simulink model "SEPIC_uniform_shading_mppt"  (R2021b)
settings: Solver=ode15s  StartTime=0.0  StopTime=1  FixedStep=1e-6  MaxStep=1e-5  RelTol=1e-3
libraries: spsDiodeLib x57, spsPVArrayLib x49, spsSeriesRLCBranchLib x6, spsMeanLib x6, spsCurrentMeasurementLib x2, spsVoltageMeasurementLib x2, simulink x1, spsIGBTDiodeLib x1, spspowerguiLib x1
settings Model: Creator=Vishal  LastModifiedBy=Vishal
settings DataIOCC: ReturnWorkspaceOutputs=off

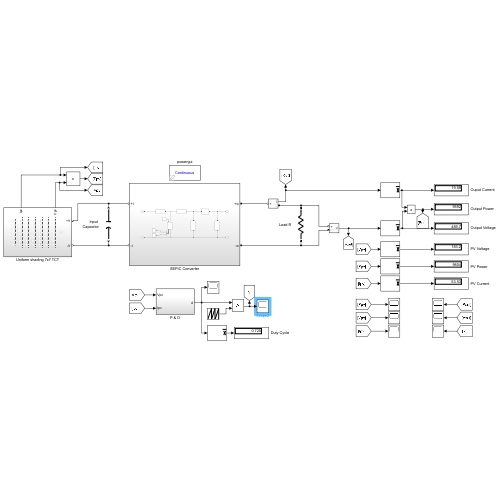
[thumbnail: Simulink's stored preview of the top-level diagram]
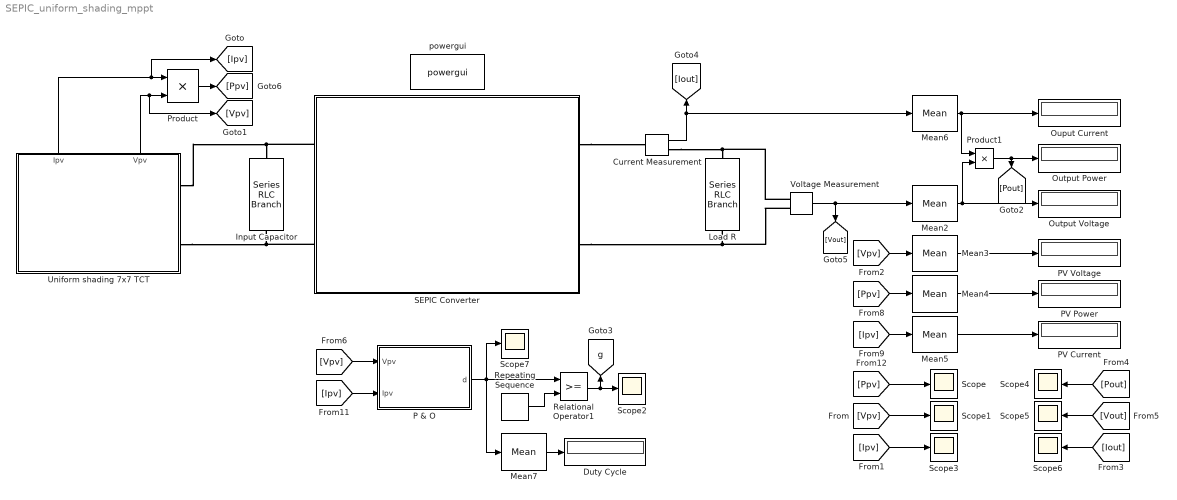
== system SEPIC_uniform_shading_mppt ==
  Current Measurement : spsCurrentMeasurementLib/Current Measurement  PhasorSimulation=off  OutputType=Complex  PSBequivalent=0
  Duty Cycle : Display
  Input Capacitor : spsSeriesRLCBranchLib/Series RLC Branch  LConnTagsString=__new0  RConnTagsString=__new0  BranchType=C  Resistance=1e-4  Inductance=1e-3  SetiL0=off  InitialCurrent=0  Capacitance=1e-3  Setx0=off  InitialVoltage=0  Measurements=None
  Load R : spsSeriesRLCBranchLib/Series RLC Branch  LConnTagsString=__new0  RConnTagsString=__new0  BranchType=R  Resistance=25  Inductance=1e-3  SetiL0=off  InitialCurrent=0  Capacitance=1e-6  Setx0=off  InitialVoltage=0  Measurements=None
  Mean{2..7} (6 alike) : spsMeanLib/Mean  Freq=10000  Vinit=0  Ts=0
  Ouput Current : Display
  Output Power : Display
  Output Voltage : Display
  P & O : Subsystem
  PV Current : Display
  PV Power : Display
  PV Voltage : Display
  Product : Product
  Product1 : Product
  Relational Operator1 : RelationalOperator  OutDataTypeStr=boolean  RndMeth=Simplest
  Repeating Sequence : simulink/Sources/Repeating Sequence  rep_seq_t=[0 1/10000]  rep_seq_y=[0 1]
  SEPIC Converter : Subsystem
  Scope{,1..7} (8 alike) : Scope
  Uniform shading 7x7 TCT : Subsystem
      settings: PortSchema="{\"entries\":[{\"content\":{\"sides\":[{\"content\":{\"connectorIds\":[]},\"type\":\"ConnectorPlacement.EquallySpacedRectSide\",\"uuid\":\"2b1d5fe4-4caa-4b35-804e-a42f89d402b6\"},{\"content\":{\"connectorIds\":[\"RConn1\",\"RConn2\"],\"side\":\"RIGHT\"},\"type\":\"ConnectorPlacement.EquallySpacedRectSide\",\"uuid\":\"1cc3aab2-123e-49fa-87cd-798c1955a822\"},{\"content\":{\"connectorIds\":[\"Out1\",\"Out2\"],\"side\":\"TOP\"},\"type\":\"ConnectorPlacement.EquallySpacedRectSide\",\"uuid\":\"89cee466-e232-436a-aff0-a5a0928aa5af\"}]},\"type\":\"ConnectorPlacement.EquallySpacedConnector\",\"uuid\":\"4c42cdc2-2679-4c70-9c6c-b31cb19848fa\"}],\"packageUris\":[\"http://schema.mathworks.com/mf0/Connector/R2020b\"],\"version\":\"1.0\"}"
  Voltage Measurement : spsVoltageMeasurementLib/Voltage Measurement  PhasorSimulation=off  OutputType=Complex  PSBequivalent=0
  powergui : spspowerguiLib/powergui  Priority=1  SimulationMode=Continuous  SampleTime=1e-6  frequency=60  Iterations=50  frequencyindice=0  Pbase=100e6  ErrMax=1e-4  UnitsV=kV  UnitsW=MW  buscounter=0  FunctionMessages=off  echomessages=off  EnableUseOfTLC=off  CurrentSourceSwitches=off  DisableSnubberDevices=off  DisableRonSwitches=off  DisableVfSwitches=off  DisplayEquations=off  AutomaticDiscreteSolvers=off  SolverType=Tustin/Backward Euler (TBE)  Interpol=off  ExternalGateDelay=off  methode=off  Ts=100  x0status=blocks  SPID=on  SwTol=0  HookPort=off  NonlinearTolerance=1e-4  nMaxIteration=100  ContinueOnMaxIteration=off  RestoreLinks=warning  ResistiveCurrentMeasurement=off  Frange=[0:2:500]  Ylog=off  Xlog=on  ShowGrid=off  save=off  variable=ZData  structure=0  ZoomFFT=off  StartTime=0.0  cycles=1  DisplayStyle=1  fundamental=60  FreqAxis=off  MaxFrequency=1000  frequencyindicesteady=1  RmsSteady=1  display=off
  tag scope: g=global
  wires:
  Product/1 -> [Ppv]
  Uniform shading 7x7 TCT/2(Vpv) -> [Vpv], Product/2
  Uniform shading 7x7 TCT/1(Ipv) -> [Ipv], Product/1
  P & O/1(d) -> Mean7/1, Scope7/1, Relational Operator1/1
  Mean7/1 -> Duty Cycle/1
  [Ppv] -> Scope/1
  Repeating Sequence/1 -> Relational Operator1/2
  [Pout] -> Scope4/1
  [Vout] -> Scope5/1
  [Ipv] -> Mean5/1
  [Iout] -> Scope6/1
  [Ipv] -> Scope3/1
  Relational Operator1/1 -> Scope2/1, [g]
  [Vpv] -> P & O/1(Vpv)
  Product1/1 -> Output Power/1, [Pout]
  [Ppv] -> Mean4/1
  [Ipv] -> P & O/2(Ipv)
  [Vpv] -> Mean3/1
  Mean6/1 -> Ouput Current/1, Product1/1
  Mean2/1 -> Output Voltage/1, Product1/2
  Mean4/1 -> PV Power/1
  Mean3/1 -> PV Voltage/1
  Mean5/1 -> PV Current/1
  Current Measurement/1 -> [Iout], Mean6/1
  [Vpv] -> Scope1/1
  Voltage Measurement/1 -> Mean2/1, [Vout]
  connections:
  Input Capacitor/LConn1 -- SEPIC Converter/LConn1 -- Uniform shading 7x7 TCT/RConn1
  Input Capacitor/RConn1 -- SEPIC Converter/LConn2 -- Uniform shading 7x7 TCT/RConn2
  Current Measurement/RConn1 -- Voltage Measurement/LConn1 -- Load R/LConn1
  Voltage Measurement/LConn2 -- SEPIC Converter/RConn2 -- Load R/RConn1
  SEPIC Converter/RConn1 -- Current Measurement/LConn1

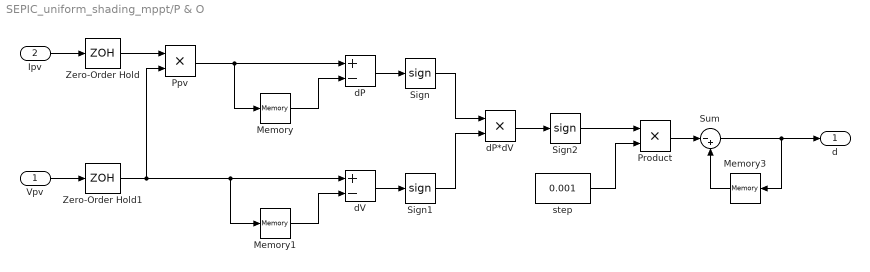
== system SEPIC_uniform_shading_mppt/P & O ==
  Vpv : Inport
  Ipv : Inport  Port=2
  Memory : Memory  InheritSampleTime=on
  Memory1 : Memory  InheritSampleTime=on
  Memory3 : Memory  InitialCondition=0.5  InheritSampleTime=on
  Ppv : Product  RndMeth=Zero
  Product : Product  RndMeth=Zero
  Sign : Signum
  Sign1 : Signum
  Sign2 : Signum
  Sum : Sum  Inputs=|-+
  Zero-Order Hold : ZeroOrderHold  SampleTime=0.002
  Zero-Order Hold1 : ZeroOrderHold  SampleTime=0.002
  dP : Sum  Inputs=+-
  dP*dV : Product  RndMeth=Zero
  dV : Sum  Inputs=+-
  step : Constant  Value=0.001
  d : Outport
  wires:
  Memory1/1 -> dV/2
  Memory/1 -> dP/2
  Vpv/1 -> Zero-Order Hold1/1
  dV/1 -> Sign1/1
  step/1 -> Product/2
  Product/1 -> Sum/1
  Sign/1 -> dP*dV/1
  Sign1/1 -> dP*dV/2
  dP*dV/1 -> Sign2/1
  Ipv/1 -> Zero-Order Hold/1
  Zero-Order Hold1/1 -> dV/1, Memory1/1, Ppv/2
  Zero-Order Hold/1 -> Ppv/1
  Ppv/1 -> Memory/1, dP/1
  dP/1 -> Sign/1
  Sign2/1 -> Product/1
  Sum/1 -> d/1, Memory3/1
  Memory3/1 -> Sum/2

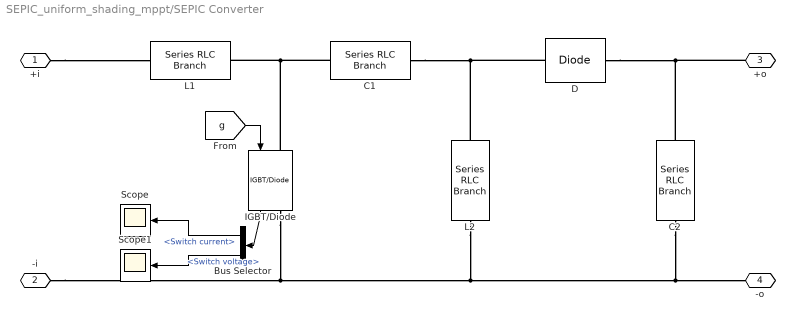
== system SEPIC_uniform_shading_mppt/SEPIC Converter ==
  Bus Selector : BusSelector  OutputSignals=Switch current,Switch voltage
  C1 : spsSeriesRLCBranchLib/Series RLC Branch  LConnTagsString=__new0  RConnTagsString=__new0  BranchType=C  Resistance=1  Inductance=1e-3  SetiL0=off  InitialCurrent=0  Capacitance=5.7143e-04  Setx0=off  InitialVoltage=0  Measurements=None
  C2 : spsSeriesRLCBranchLib/Series RLC Branch  LConnTagsString=__new0  RConnTagsString=__new0  BranchType=C  Resistance=1  Inductance=1e-3  SetiL0=off  InitialCurrent=0  Capacitance=0.0029  Setx0=off  InitialVoltage=0  Measurements=None
  D : spsDiodeLib/Diode  Ron=0.001  Lon=0  Vf=0  IC=0  UseSnubber=0  Rs=500  Cs=250e-9  Measurements=off
  IGBT/Diode : spsIGBTDiodeLib/IGBT//Diode  Ron=1e-3  Rs=1e5  Cs=inf  Measurements=on
  L1 : spsSeriesRLCBranchLib/Series RLC Branch  LConnTagsString=__new0  RConnTagsString=__new0  BranchType=L  Resistance=1  Inductance=0.0143  SetiL0=off  InitialCurrent=0  Capacitance=1e-6  Setx0=off  InitialVoltage=0  Measurements=None
  L2 : spsSeriesRLCBranchLib/Series RLC Branch  LConnTagsString=__new0  RConnTagsString=__new0  BranchType=L  Resistance=1  Inductance=0.0107  SetiL0=off  InitialCurrent=0  Capacitance=1e-6  Setx0=off  InitialVoltage=0  Measurements=None
  Scope : Scope
  Scope1 : Scope
  +i : PMIOPort  Side=Left
  -i : PMIOPort  Port=2  Side=Left
  +o : PMIOPort  Port=3  Side=Right
  -o : PMIOPort  Port=4  Side=Right
  wires:
  [g] -> IGBT/Diode/1
  Bus Selector/1 -> Scope/1  "<Switch current>"
  IGBT/Diode/1 -> Bus Selector/1
  Bus Selector/2 -> Scope1/1  "<Switch voltage>"
  connections:
  C1/LConn1 -- L1/RConn1 -- IGBT/Diode/LConn1
  C1/RConn1 -- L2/RConn1 -- D/LConn1
  C2/LConn1 -- D/RConn1 -- +o/RConn1
  +i/RConn1 -- L1/LConn1
  -i/RConn1 -- L2/LConn1 -- -o/RConn1 -- C2/RConn1 -- IGBT/Diode/RConn1

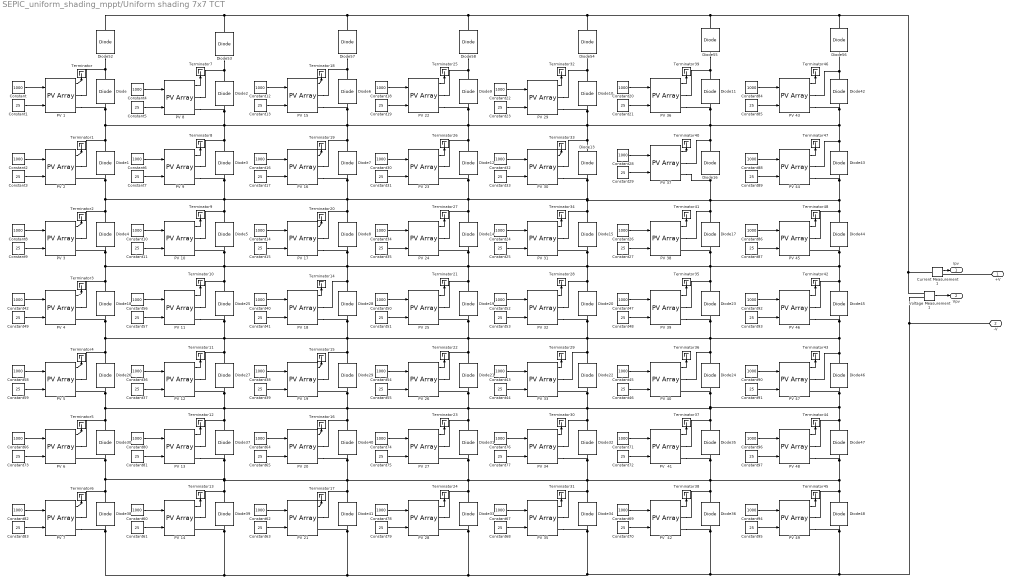
== system SEPIC_uniform_shading_mppt/Uniform shading 7x7 TCT ==
  Constant{,2,4,6,8,10,12,14,16,18,20,22,24,26,28,30,32,34,36,38,40,42..43,45,47,50,52,54,56,58,60,62,64,66..67,69,71,74,76,78,80,82,84,86,88,90,92,94,96} (49 alike) : Constant  Value=1000
  Constant{1,3,5,7,9,11,13,15,17,19,21,23,25,27,29,31,33,35,37,39,41,44,46,48..49,51,53,55,57,59,61,63,65,68,70,72..73,75,77,79,81,83,85,87,89,91,93,95,97} (49 alike) : Constant  Value=25
  Current Measurement1 : spsCurrentMeasurementLib/Current Measurement  PhasorSimulation=off  OutputType=Complex  PSBequivalent=0
  Diode{,1..48,52..58} (56 alike) : spsDiodeLib/Diode  Ron=0.001  Lon=0  Vf=0  IC=0  UseSnubber=0  Rs=500  Cs=250e-9  Measurements=off
  PV  41 : spsPVArrayLib/PV Array  Npar=1  Nser=1  PlotType=array @ 1000 W/m2 & specified temperatures  S_vec="[ 1000  500  100 ]"  Temp_C_vec="[ 45 25  ]"  ModuleName=Kyocera Solar KC200GT  PlotWhenSelected=off  Pm=200.143  Ncell=54  Voc=32.9  Isc=8.21  Vm=26.3  Im=7.61  beta_Voc_pc=-0.355  alpha_Isc_pc=0.06  beta_Voc=-0.11679  alpha_Isc=0.004926  IL=8.2288  I0=2.3234e-10  nI=0.97734  Rsh=150.6844  Rs=0.34484  RobustModel=off  RobustCellTemperature=313.3991  BAL=on  Tc=1e-6  Tfilter=5e-5
  PV  42 : spsPVArrayLib/PV Array  Npar=1  Nser=1  PlotType=array @ 1000 W/m2 & specified temperatures  S_vec="[ 1000  500  100 ]"  Temp_C_vec="[ 45 25  ]"  ModuleName=Kyocera Solar KC200GT  PlotWhenSelected=off  Pm=200.143  Ncell=54  Voc=32.9  Isc=8.21  Vm=26.3  Im=7.61  beta_Voc_pc=-0.355  alpha_Isc_pc=0.06  beta_Voc=-0.11679  alpha_Isc=0.004926  IL=8.2288  I0=2.3234e-10  nI=0.97734  Rsh=150.6844  Rs=0.34484  RobustModel=off  RobustCellTemperature=313.3991  BAL=on  Tc=1e-6  Tfilter=5e-5
  PV {1..40,43..49} (47 alike) : spsPVArrayLib/PV Array  Npar=1  Nser=1  PlotType=array @ 1000 W/m2 & specified temperatures  S_vec="[ 1000  500  100 ]"  Temp_C_vec="[ 45 25  ]"  ModuleName=Kyocera Solar KC200GT  PlotWhenSelected=off  Pm=200.143  Ncell=54  Voc=32.9  Isc=8.21  Vm=26.3  Im=7.61  beta_Voc_pc=-0.355  alpha_Isc_pc=0.06  beta_Voc=-0.11679  alpha_Isc=0.004926  IL=8.2288  I0=2.3234e-10  nI=0.97734  Rsh=150.6844  Rs=0.34484  RobustModel=off  RobustCellTemperature=313.3991  BAL=on  Tc=1e-6  Tfilter=5e-5
  Terminator{,1..48} (49 alike) : Terminator
  Voltage Measurement1 : spsVoltageMeasurementLib/Voltage Measurement  PhasorSimulation=off  OutputType=Complex  PSBequivalent=0
  +V : PMIOPort  Side=Right
  -V : PMIOPort  Port=2  Side=Right
  Ipv : Outport
  Vpv : Outport  Port=2
  wires:
  Constant91/1 -> PV 47/2
  PV 20/1 -> Terminator16/1
  Constant93/1 -> PV 46/2
  PV 23/1 -> Terminator26/1
  Constant87/1 -> PV 45/2
  Constant46/1 -> PV 40/2
  PV 49/1 -> Terminator45/1
  PV 47/1 -> Terminator43/1
  PV 48/1 -> Terminator44/1
  Constant60/1 -> PV 14/1
  Constant70/1 -> PV  42/2
  Constant1/1 -> PV 1/2
  Constant61/1 -> PV 14/2
  PV  41/1 -> Terminator37/1
  PV 11/1 -> Terminator10/1
  Constant8/1 -> PV 3/1
  Constant39/1 -> PV 19/2
  Constant47/1 -> PV 39/1
  Constant73/1 -> PV 6/2
  Constant25/1 -> PV 31/2
  Constant33/1 -> PV 30/2
  PV 30/1 -> Terminator33/1
  PV 45/1 -> Terminator48/1
  Constant13/1 -> PV 15/2
  Constant86/1 -> PV 45/1
  Constant6/1 -> PV 9/1
  PV 27/1 -> Terminator23/1
  Constant82/1 -> PV 7/1
  PV 22/1 -> Terminator25/1
  Constant58/1 -> PV 5/1
  PV 35/1 -> Terminator31/1
  Constant74/1 -> PV 27/1
  PV 1/1 -> Terminator/1
  Constant32/1 -> PV 30/1
  Constant55/1 -> PV 26/2
  PV  42/1 -> Terminator38/1
  PV 28/1 -> Terminator24/1
  Constant65/1 -> PV 20/2
  Constant50/1 -> PV 25/1
  Constant40/1 -> PV 18/1
  Constant37/1 -> PV 12/2
  Constant90/1 -> PV 47/1
  PV 7/1 -> Terminator6/1
  PV 6/1 -> Terminator5/1
  Constant/1 -> PV 1/1
  PV 36/1 -> Terminator39/1
  PV 29/1 -> Terminator32/1
  PV 2/1 -> Terminator1/1
  Constant94/1 -> PV 49/1
  Constant22/1 -> PV 29/1
  Constant38/1 -> PV 19/1
  Constant16/1 -> PV 16/1
  PV 46/1 -> Terminator42/1
  PV 9/1 -> Terminator8/1
  Constant48/1 -> PV 39/2
  PV 10/1 -> Terminator9/1
  Constant88/1 -> PV 44/1
  Constant11/1 -> PV 10/2
  Constant54/1 -> PV 26/1
  Constant56/1 -> PV 11/1
  Constant69/1 -> PV  42/1
  PV 44/1 -> Terminator47/1
  Constant20/1 -> PV 36/1
  PV 34/1 -> Terminator30/1
  Constant83/1 -> PV 7/2
  Constant27/1 -> PV 38/2
  PV 43/1 -> Terminator46/1
  Constant23/1 -> PV 29/2
  Constant31/1 -> PV 23/2
  Constant9/1 -> PV 3/2
  Constant28/1 -> PV 37/1
  PV 4/1 -> Terminator3/1
  Constant30/1 -> PV 23/1
  Constant79/1 -> PV 28/2
  Constant49/1 -> PV 4/2
  PV 12/1 -> Terminator11/1
  Constant5/1 -> PV 8/2
  PV 18/1 -> Terminator14/1
  Constant96/1 -> PV 48/1
  PV 39/1 -> Terminator35/1
  Constant97/1 -> PV 48/2
  Constant89/1 -> PV 44/2
  Constant53/1 -> PV 32/2
  Constant2/1 -> PV 2/1
  Constant64/1 -> PV 20/1
  Constant72/1 -> PV  41/2
  PV 15/1 -> Terminator18/1
  Constant26/1 -> PV 38/1
  PV 38/1 -> Terminator41/1
  Constant45/1 -> PV 40/1
  PV 8/1 -> Terminator7/1
  PV 17/1 -> Terminator20/1
  Constant57/1 -> PV 11/2
  PV 14/1 -> Terminator13/1
  Constant43/1 -> PV 33/1
  Constant19/1 -> PV 22/2
  PV 24/1 -> Terminator27/1
  Constant35/1 -> PV 24/2
  Constant59/1 -> PV 5/2
  Constant84/1 -> PV 43/1
  PV 32/1 -> Terminator28/1
  Constant67/1 -> PV 35/1
  PV 40/1 -> Terminator36/1
  PV 19/1 -> Terminator15/1
  PV 33/1 -> Terminator29/1
  PV 13/1 -> Terminator12/1
  Constant17/1 -> PV 16/2
  Constant10/1 -> PV 10/1
  Voltage Measurement1/1 -> Vpv/1
  Constant21/1 -> PV 36/2
  PV 5/1 -> Terminator4/1
  Constant66/1 -> PV 6/1
  Constant85/1 -> PV 43/2
  Constant51/1 -> PV 25/2
  Constant52/1 -> PV 32/1
  Constant81/1 -> PV 13/2
  Constant36/1 -> PV 12/1
  Constant44/1 -> PV 33/2
  Constant42/1 -> PV 4/1
  PV 16/1 -> Terminator19/1
  PV 26/1 -> Terminator22/1
  Constant14/1 -> PV 17/1
  PV 31/1 -> Terminator34/1
  PV 3/1 -> Terminator2/1
  Constant4/1 -> PV 8/1
  Constant41/1 -> PV 18/2
  Constant92/1 -> PV 46/1
  Constant80/1 -> PV 13/1
  Constant63/1 -> PV 21/2
  Constant3/1 -> PV 2/2
  Constant77/1 -> PV 34/2
  Constant24/1 -> PV 31/1
  PV 37/1 -> Terminator40/1
  Constant71/1 -> PV  41/1
  Constant95/1 -> PV 49/2
  Constant29/1 -> PV 37/2
  Constant34/1 -> PV 24/1
  Constant76/1 -> PV 34/1
  Constant75/1 -> PV 27/2
  Constant15/1 -> PV 17/2
  Constant78/1 -> PV 28/1
  PV 25/1 -> Terminator21/1
  Constant18/1 -> PV 22/1
  Constant68/1 -> PV 35/2
  Constant7/1 -> PV 9/2
  Constant12/1 -> PV 15/1
  Constant62/1 -> PV 21/1
  PV 21/1 -> Terminator17/1
  Current Measurement1/1 -> Ipv/1
  connections:
  PV 7/RConn1 -- PV 13/RConn2 -- Diode37/LConn1 -- PV 20/RConn2 -- Diode40/LConn1 -- PV 28/RConn1 -- Diode33/RConn1 -- PV 34/RConn2 -- Diode32/LConn1 -- PV  41/RConn2 -- Diode35/LConn1 -- Diode47/LConn1 -- PV 48/RConn2 -- Diode48/RConn1 -- PV 49/RConn1 -- Diode36/RConn1 -- PV  42/RConn1 -- Diode34/RConn1 -- PV 35/RConn1 -- PV 27/RConn2 -- Diode31/LConn1 -- Diode41/RConn1 -- PV 21/RConn1 -- Diode39/RConn1 -- PV 14/RConn1 -- Diode30/LConn1 -- PV 6/RConn2 -- Diode38/RConn1
  PV 22/RConn1 -- Diode9/RConn1 -- Diode58/LConn1
  Diode54/RConn1 -- Diode53/RConn1 -- Diode52/RConn1 -- Diode57/RConn1 -- Diode58/RConn1 -- Diode55/RConn1 -- Current Measurement1/LConn1 -- Voltage Measurement1/LConn1 -- Diode56/RConn1
  Diode4/LConn1 -- Diode18/RConn1 -- PV 4/RConn1 -- PV 11/RConn1 -- Diode25/RConn1 -- PV 18/RConn1 -- Diode28/RConn1 -- PV 39/RConn1 -- Diode23/RConn1 -- Diode45/RConn1 -- PV 46/RConn1 -- Diode44/LConn1 -- PV 45/RConn2 -- Diode17/LConn1 -- PV 38/RConn2 -- Diode15/LConn1 -- PV 31/RConn2 -- PV 32/RConn1 -- Diode20/RConn1 -- PV 25/RConn1 -- Diode19/RConn1 -- PV 24/RConn2 -- Diode14/LConn1 -- Diode8/LConn1 -- PV 17/RConn2 -- Diode5/LConn1 -- PV 10/RConn2 -- PV 3/RConn2
  Voltage Measurement1/LConn2 -- -V/RConn1 -- Diode48/LConn1 -- PV 49/RConn2 -- Diode33/LConn1 -- PV 28/RConn2 -- Diode41/LConn1 -- PV 21/RConn2 -- Diode39/LConn1 -- PV 14/RConn2 -- Diode38/LConn1 -- PV 7/RConn2 -- Diode34/LConn1 -- PV 35/RConn2 -- Diode36/LConn1 -- PV  42/RConn2
  PV 15/RConn1 -- Diode6/RConn1 -- Diode57/LConn1
  PV 1/RConn1 -- Diode/RConn1 -- Diode52/LConn1
  PV 8/RConn1 -- Diode2/RConn1 -- Diode53/LConn1
  PV 29/RConn1 -- Diode10/RConn1 -- Diode54/LConn1
  PV 5/RConn2 -- Diode30/RConn1 -- PV 6/RConn1 -- Diode27/LConn1 -- PV 12/RConn2 -- PV 13/RConn1 -- Diode37/RConn1 -- PV 19/RConn2 -- Diode29/LConn1 -- Diode40/RConn1 -- PV 20/RConn1 -- Diode21/LConn1 -- PV 26/RConn2 -- PV 27/RConn1 -- Diode31/RConn1 -- Diode46/LConn1 -- PV 47/RConn2 -- Diode47/RConn1 -- PV 48/RConn1 -- Diode24/LConn1 -- PV 40/RConn2 -- PV  41/RConn1 -- Diode35/RConn1 -- Diode22/LConn1 -- PV 33/RConn2 -- PV 34/RConn1 -- Diode32/RConn1 -- Diode26/LConn1
  PV 43/RConn1 -- Diode56/LConn1 -- Diode42/RConn1
  PV 3/RConn1 -- Diode4/RConn1 -- Diode8/RConn1 -- PV 17/RConn1 -- PV 23/RConn2 -- Diode12/LConn1 -- Diode13/LConn1 -- PV 30/RConn2 -- PV 37/RConn2 -- Diode16/LConn1 -- Diode43/LConn1 -- PV 44/RConn2 -- Diode44/RConn1 -- PV 45/RConn1 -- Diode17/RConn1 -- PV 38/RConn1 -- PV 31/RConn1 -- Diode15/RConn1 -- PV 24/RConn1 -- Diode14/RConn1 -- PV 16/RConn2 -- Diode7/LConn1 -- Diode5/RConn1 -- PV 10/RConn1 -- PV 9/RConn2 -- Diode3/LConn1 -- PV 2/RConn2 -- Diode1/LConn1
  PV 5/RConn1 -- PV 19/RConn1 -- Diode29/RConn1 -- PV 25/RConn2 -- Diode19/LConn1 -- Diode20/LConn1 -- PV 32/RConn2 -- Diode23/LConn1 -- PV 39/RConn2 -- PV 46/RConn2 -- Diode45/LConn1 -- PV 47/RConn1 -- Diode46/RConn1 -- Diode24/RConn1 -- PV 40/RConn1 -- Diode22/RConn1 -- PV 33/RConn1 -- PV 26/RConn1 -- Diode21/RConn1 -- Diode28/LConn1 -- PV 18/RConn2 -- Diode27/RConn1 -- PV 12/RConn1 -- PV 11/RConn2 -- Diode25/LConn1 -- PV 4/RConn2 -- Diode18/LConn1 -- Diode26/RConn1
  PV 1/RConn2 -- Diode1/RConn1 -- PV 2/RConn1 -- PV 8/RConn2 -- Diode2/LConn1 -- Diode10/LConn1 -- PV 29/RConn2 -- Diode11/LConn1 -- PV 36/RConn2 -- PV 43/RConn2 -- Diode42/LConn1 -- PV 44/RConn1 -- Diode43/RConn1 -- PV 37/RConn1 -- Diode16/RConn1 -- PV 30/RConn1 -- Diode13/RConn1 -- Diode12/RConn1 -- PV 23/RConn1 -- PV 22/RConn2 -- Diode9/LConn1 -- Diode6/LConn1 -- PV 15/RConn2 -- PV 16/RConn1 -- Diode7/RConn1 -- PV 9/RConn1 -- Diode3/RConn1 -- Diode/LConn1
  +V/RConn1 -- Current Measurement1/RConn1
  PV 36/RConn1 -- Diode11/RConn1 -- Diode55/LConn1
